simulink model "Problem1"  (R2020a)
settings: Solver=VariableStepAuto  StartTime=0.0  StopTime=10.0  RelTol=1e-3
settings Model: Creator=tanu  LastModifiedBy=tanu

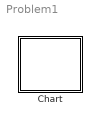
== system Problem1 ==
  Chart : Stateflow chart  TreatAsAtomicUnit=on

== stateflow chart Problem1/Chart ==
  state No_coins
  state Rupee_5
  state Rupee_10
  (default) -> No_coins
  No_coins -> Rupee_5 [order 1] : [coin==1]{soda=0}
  Rupee_5 -> No_coins [order 2] : [coin==2]{soda=1}
  Rupee_10 -> No_coins [order 1] : [coin==1]{soda=1}
  No_coins -> Rupee_10 [order 2] : [coin==2]{soda=0}
  Rupee_10 -> Rupee_5 [order 2] : [coin==2]{soda=1}
  Rupee_5 -> Rupee_10 [order 1] : [coin==1]{soda=0}
